simulink model "Exemplu_figura6"  (R2016a)
settings: Solver=VariableStepAuto  StartTime=0.0  StopTime=100  RelTol=1e-3
undefined symbols (not defined in the file): m
settings Model: Creator=Cristina  LastModifiedBy=Cristina

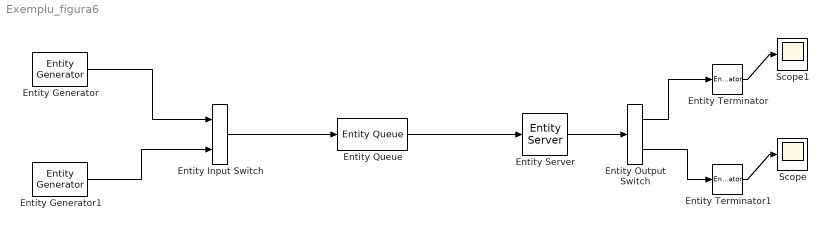
== system Exemplu_figura6 ==
  Entity Input Switch : EntityInputSwitch  InputPortMessageModes=m,m  OutputPortMessageModes=m
  Entity Output Switch : EntityOutputSwitch  InputPortMessageModes=m  OutputPortMessageModes=m,m  SwitchingCriterion=From attribute  SwitchAttributeName=prt
  Entity Generator : EntityGenerator  OutputPortMessageModes=m  TimeSource=MATLAB action  IntergenerationTimeAction=|  GenerateAction=|  AttributeName=ServiceTime|prt  AttributeInitialValue=1|1  EntityType=Structured  EntityTypeName=Entity
      IntergenerationTimeAction=|
      | persistent init
      | if (isempty(init))
      |     rng(113);
      |     init = true;
      | end
      | dt = exprnd(0.5);
      GenerateAction=|
      | persistent st
      | if(isempty(st))
      |     rng(465);
      |     st = true;
      | end
      | entity.ServiceTime = exprnd(0.3);
  Entity Generator1 : EntityGenerator  OutputPortMessageModes=m  TimeSource=MATLAB action  IntergenerationTimeAction=|  AttributeName=ServiceTime|prt  AttributeInitialValue=1|2  EntityType=Structured  EntityTypeName=Entity
      | persistent init
      | if (isempty(init))
      |     rng(113);
      |     init = true;
      | end
      | dt = exprnd(0.5);
  Entity Queue : EntityQueue  InputPortMessageModes=m  OutputPortMessageModes=m
      settings: OutputPortMap=o5
  Entity Server : EntityServer  InputPortMessageModes=m  OutputPortMessageModes=m  Capacity=1  ServiceTimeSource=Attribute
  Entity Terminator : EntityTerminator  InputPortMessageModes=m  NumberEntitiesArrived=on
      settings: OutputPortMap=o0
  Entity Terminator1 : EntityTerminator  InputPortMessageModes=m  NumberEntitiesArrived=on
      settings: OutputPortMap=o0
  Scope : Scope
  Scope1 : Scope
  wires:
  Entity Input Switch/1 -> Entity Queue/1
  Entity Generator/1 -> Entity Input Switch/1
  Entity Generator1/1 -> Entity Input Switch/2
  Entity Queue/1 -> Entity Server/1
  Entity Server/1 -> Entity Output Switch/1
  Entity Output Switch/1 -> Entity Terminator/1
  Entity Output Switch/2 -> Entity Terminator1/1
  Entity Terminator1/1 -> Scope/1
  Entity Terminator/1 -> Scope1/1
